simulink model "Antilock_brake_system"  (R2020b)
settings: Solver=VariableStepAuto  StartTime=0.0  StopTime=10.0  RelTol=1e-3
values from neighbouring files (symbols this model uses):
  ctrl = 1    [data_abs.m]
  g = 32.18    [data_abs.m]
  m = 50    [data_abs.m]
  mu = [0 .4 .8 .97 1.0 .98 .96 .94 .92 .9 .88 .855 .83 .81 .79 .77 .75 .73 .72 .71 .7]    [data_abs.m]
  Rr = 15/12    (= 1.25)    [data_abs.m]
  slip = (0:.05:1.0)    [data_abs.m]
  v0 = 88    [data_abs.m]
settings Model: Creator=153  LastModifiedBy=153
settings DebuggingCC: AlgebraicLoopMsg=none  ArtificialAlgebraicLoopMsg=none

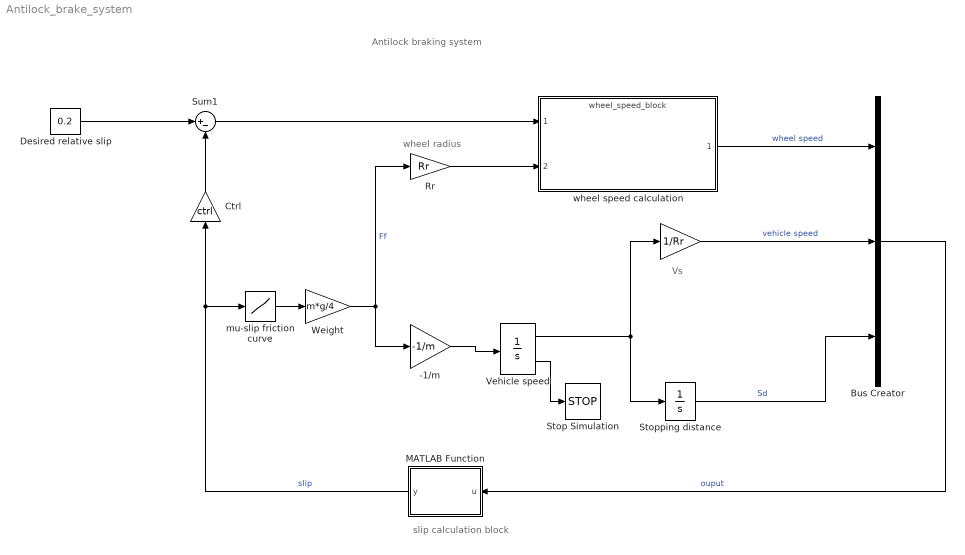
== system Antilock_brake_system ==
  note: slip calculation block
  note: Vs
  note: wheel radius
  note: Antilock braking system
  " " : Gain  Gain=1/Rr  SaturateOnIntegerOverflow=on  OutDataTypeStr=Inherit: Same as input  ParamDataTypeStr=Inherit: Same as input
  -1/m : Gain  Gain=-1/m  SaturateOnIntegerOverflow=on  OutDataTypeStr=Inherit: Same as input  ParamDataTypeStr=Inherit: Same as input
  Bus Creator : BusCreator  Inputs=3
  Ctrl : Gain  Gain=ctrl  SaturateOnIntegerOverflow=on  OutDataTypeStr=Inherit: Same as input  ParamDataTypeStr=Inherit: Same as input
  Desired relative slip : Constant  Value=0.2
  MATLAB Function : MATLAB Function  TreatAsAtomicUnit=on
  Rr : Gain  Gain=Rr  SaturateOnIntegerOverflow=on  OutDataTypeStr=Inherit: Same as input  ParamDataTypeStr=Inherit: Same as input
  Stop Simulation : Stop
  Stopping distance : Integrator  UpperSaturationLimit=1000  LowerSaturationLimit=0
  Sum1 : Sum  Inputs=|+-  InputSameDT=on  SaturateOnIntegerOverflow=on  OutDataTypeStr=Inherit: Same as first input
  Vehicle speed : Integrator  InitialCondition=v0  LimitOutput=on  UpperSaturationLimit=1000  LowerSaturationLimit=0  ShowSaturationPort=on
  Weight : Gain  Gain=m*g/4  SaturateOnIntegerOverflow=on  OutDataTypeStr=Inherit: Same as input  ParamDataTypeStr=Inherit: Same as input
  mu-slip friction curve : Lookup_n-D  NumberOfTableDimensions=1  BreakpointsForDimension1=slip  Table=mu  SaturateOnIntegerOverflow=on  InputSameDT=on
  wheel speed calculation : ModelReference  ModelNameDialog=wheel_speed_block  SimulationMode=Normal  ModelReferenceVersion=1.2
  wires:
  Sum1/1 -> wheel speed calculation/1
  Vehicle speed/1 -> Stopping distance/1, " "/1
  Rr/1 -> wheel speed calculation/2
  " "/1 -> Bus Creator/2  "vehicle speed"
  mu-slip friction curve/1 -> Weight/1
  wheel speed calculation/1 -> Bus Creator/1  "wheel speed"
  Desired relative slip/1 -> Sum1/1
  Ctrl/1 -> Sum1/2
  Weight/1 -> -1/m/1, Rr/1  "Ff"
  -1/m/1 -> Vehicle speed/1
  Stopping distance/1 -> Bus Creator/3  "Sd"
  MATLAB Function/1(y) -> mu-slip friction curve/1, Ctrl/1  "slip"
  Bus Creator/1 -> MATLAB Function/1(u)  "ouput"
  Vehicle speed/2 -> Stop Simulation/1

== matlab function Antilock_brake_system/MATLAB Function ==
  data: u input; y output
function y = fcn(u)
y = 1.0 - u(1)/(u(2) + (u(2)==0)*eps);
